simulink model "chap3_5"  (Simulink 5.0)
settings: Solver=ode45  StartTime=0.0  StopTime=3  RelTol=1e-3
libraries: fuzblock x1
settings Model: ExtModeTrigMode=oneshot  ExtModeArmWhenConnect=off  LimitDataPoints=off  BooleanDataType=off

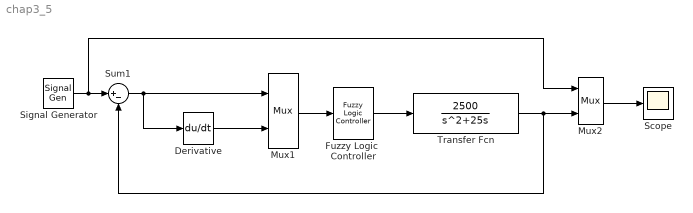
== system chap3_5 ==
  Derivative : Derivative
  Fuzzy Logic  Controller : fuzblock/Fuzzy Logic  Controller  fis=a2
  Mux1 : Mux  Inputs=2
  Mux2 : Mux  Inputs=2
  Scope : Scope
      settings: TimeRange=1  YMin=0.425  YMax=1
  Signal Generator : SignalGenerator
  Sum1 : Sum  Inputs=|+-  SaturateOnIntegerOverflow=on  InputSameDT=on
  Transfer Fcn : TransferFcn  Numerator=[2500]  Denominator=[1 25 0]
  wires:
  Mux1/1 -> Fuzzy Logic  Controller/1
  Mux2/1 -> Scope/1
  Sum1/1 -> Mux1/1, Derivative/1
  Signal Generator/1 -> Sum1/1, Mux2/1
  Fuzzy Logic  Controller/1 -> Transfer Fcn/1
  Transfer Fcn/1 -> Mux2/2, Sum1/2
  Derivative/1 -> Mux1/2
